simulink model "Catch_the_ball_gaming_machine"  (R2019a)
settings: Solver=VariableStepAuto  StartTime=0.0  StopTime=10.0  RelTol=1e-3
libraries: arduinolib x17
settings Model: Creator=Subhau  LastModifiedBy=Subhau

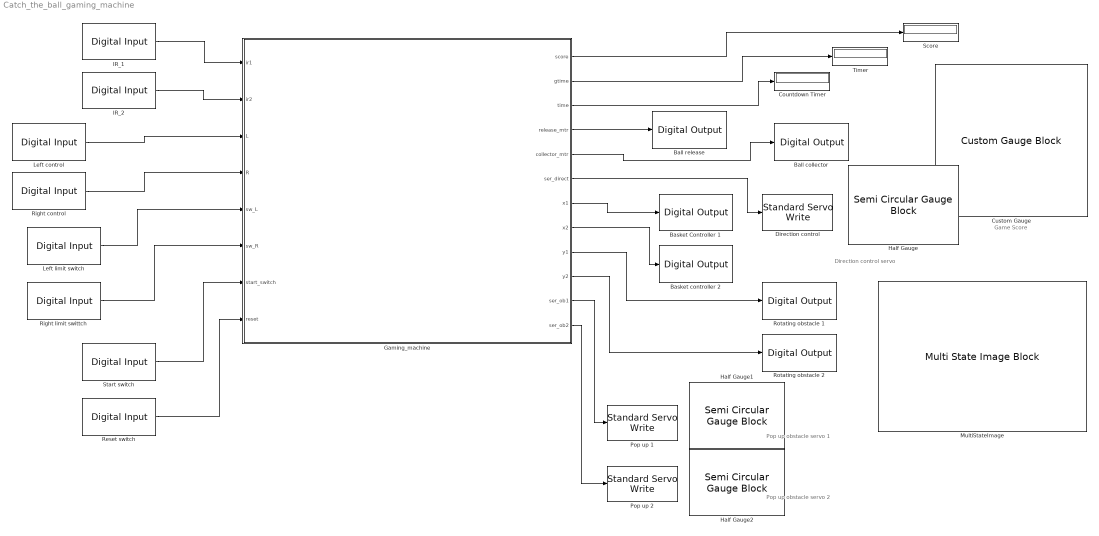
== system Catch_the_ball_gaming_machine ==
  note: Direction control servo
  note: Pop up obstacle servo 1
  note: Pop up obstacle servo 2
  note: Game Score
  Ball collector : arduinolib/Digital Output  pinNumber=20  blockPlatform=arduino
  Ball release : arduinolib/Digital Output  pinNumber=21  blockPlatform=arduino
  Basket Controller 1 : arduinolib/Digital Output  pinNumber=22  blockPlatform=arduino
  Basket controller 2 : arduinolib/Digital Output  pinNumber=23  blockPlatform=arduino
  Countdown Timer : Display
  Custom Gauge : CustomGaugeBlock  NeedleImage=data:image/svg+xml;base64,PD94bWwgdmVyc2lvbj0iMS4wIiBlbmNvZGluZz0idXRmLTgiPz4KPCEtLSBHZW5lcmF0b3I6IEFkb2JlIElsbHVzdHJhdG9yIDE5LjIuMSwgU1ZHIEV4cG9ydCBQbHVnLUluIC4gU1ZHIFZlcnNpb246IDYuMDAgQnVpbGQgMCkgIC0tPgo8c3ZnIHZlcnNpb249IjEuMSIgeG1sbnM9Imh0dHA6Ly93d3cudzMub3JnLzIwMDAvc3ZnIiB4bWxuczp4bGluaz0iaHR0cDovL3d3dy53My5vcmcvMTk5OS94bGluayIgeD0iMHB4IiB5PSIwcHgiCgkgdmlld0JveD0iMCAwIDIwMCA1MCIgc3R5bGU9ImVuYWJsZS1iYWNrZ3JvdW5kOm5ldyAw ...(+9940 chars)  NeedleXPos=0.3802298124325669  NeedleYPos=0.48117305677424654  NeedleHeight=0.11602152693163792  NeedleWidth=0.1911368983686954  NeedleInitialRotation=-59.94322499147643  BackgroundImage=data:image/svg+xml;base64,PD94bWwgdmVyc2lvbj0iMS4wIiBlbmNvZGluZz0iVVRGLTgiIHN0YW5kYWxvbmU9Im5vIj8+CjwhLS0gR2VuZXJhdG9yOiBBZG9iZSBJbGx1c3RyYXRvciAxOS4yLjEsIFNWRyBFeHBvcnQgUGx1Zy1JbiAuIFNWRyBWZXJzaW9uOiA2LjAwIEJ1aWxkIDApICAtLT4KCjxzdmcKICAgeG1sbnM6ZGM9Imh0dHA6Ly9wdXJsLm9yZy9kYy9lbGVtZW50cy8xLjEvIgogICB4bWxuczpjYz0iaHR0cDovL2NyZWF0aXZlY29tbW9ucy5vcmcvbnMjIgogICB4bWxuczpyZGY9Imh0dHA6Ly93d3cudzMub3JnLzE5OTkvMDIvMjItcmRmLXN5bnRh ...(+9660 chars)  GaugeMax=1000  GaugeArcDefined=true  GaugeArcRadius=0.1358563990074277  GaugeArcStrokeWidth=0.03972965542329953  GaugeArcRotation=240.5385250290321  GaugeArcRatio=0.8333333333333  GaugeArcTransparency=0  ValueArcColor=#1759b0  GaugeTickColor=#faf5c8  TickInterval=200  ScaleColorsJSON=[]  fixedAspectRatio=on
  Direction control : arduinolib/Standard Servo Write  pinNumber=2  ServoIndex=0  blockPlatform=ARDUINO
      settings: SourceProductName=Simulink Support Package for Arduino Hardware
  Gaming_machine : Stateflow chart  BlockKeywords=__PRM__SERIALIZED__DATA__:Stateflow Chart,Stateflow Diagram  TreatAsAtomicUnit=on
  Half Gauge : SemiCircularGaugeBlock  ScaleMax=180  TickInterval=30
  Half Gauge1 : SemiCircularGaugeBlock  ScaleMax=180  TickInterval=30
  Half Gauge2 : SemiCircularGaugeBlock  ScaleMax=180  TickInterval=30
  IR_1 : arduinolib/Digital Input  pinNumber=4  sampleTime=0.1  blockPlatform=arduino
      settings: SourceProductName=Simulink Support Package for Arduino Hardware
  IR_2 : arduinolib/Digital Input  pinNumber=5  sampleTime=0.1  blockPlatform=arduino
      settings: SourceProductName=Simulink Support Package for Arduino Hardware
  Left control : arduinolib/Digital Input  pinNumber=6  sampleTime=0.1  blockPlatform=arduino
      settings: SourceProductName=Simulink Support Package for Arduino Hardware
  Left limit switch : arduinolib/Digital Input  pinNumber=8  sampleTime=0.1  blockPlatform=arduino
      settings: SourceProductName=Simulink Support Package for Arduino Hardware
  MultiStateImage : MultiStateImageBlock
  Pop up 1 : arduinolib/Standard Servo Write  pinNumber=45  ServoIndex=1  blockPlatform=ARDUINO
      settings: SourceProductName=Simulink Support Package for Arduino Hardware
  Pop up 2 : arduinolib/Standard Servo Write  pinNumber=3  ServoIndex=2  blockPlatform=ARDUINO
      settings: SourceProductName=Simulink Support Package for Arduino Hardware
  Reset switch : arduinolib/Digital Input  pinNumber=11  sampleTime=0.1  blockPlatform=arduino
      settings: SourceProductName=Simulink Support Package for Arduino Hardware
  Right control : arduinolib/Digital Input  pinNumber=7  sampleTime=0.1  blockPlatform=arduino
      settings: SourceProductName=Simulink Support Package for Arduino Hardware
  Right limit swittch : arduinolib/Digital Input  pinNumber=9  sampleTime=0.1  blockPlatform=arduino
      settings: SourceProductName=Simulink Support Package for Arduino Hardware
  Rotating obstacle 1 : arduinolib/Digital Output  pinNumber=24  blockPlatform=arduino
  Rotating obstacle 2 : arduinolib/Digital Output  pinNumber=25  blockPlatform=arduino
  Score : Display
  Start switch : arduinolib/Digital Input  pinNumber=10  sampleTime=0.1  blockPlatform=arduino
      settings: SourceProductName=Simulink Support Package for Arduino Hardware
  Timer : Display
  wires:
  Reset switch/1 -> Gaming_machine/8(reset)
  Gaming_machine/2(gtime) -> Timer/1
  Left control/1 -> Gaming_machine/3(L)
  IR_1/1 -> Gaming_machine/1(ir1)
  Right control/1 -> Gaming_machine/4(R)
  Gaming_machine/1(score) -> Score/1
  Left limit switch/1 -> Gaming_machine/5(sw_L)
  Gaming_machine/3(time) -> Countdown Timer/1
  IR_2/1 -> Gaming_machine/2(ir2)
  Start switch/1 -> Gaming_machine/7(start_switch)
  Right limit swittch/1 -> Gaming_machine/6(sw_R)
  Gaming_machine/8(x2) -> Basket controller 2/1
  Gaming_machine/6(ser_direct) -> Direction control/1
  Gaming_machine/9(y1) -> Rotating obstacle 1/1
  Gaming_machine/4(release_mtr) -> Ball release/1
  Gaming_machine/11(ser_ob1) -> Pop up 1/1
  Gaming_machine/12(ser_ob2) -> Pop up 2/1
  Gaming_machine/7(x1) -> Basket Controller 1/1
  Gaming_machine/5(collector_mtr) -> Ball collector/1
  Gaming_machine/10(y2) -> Rotating obstacle 2/1

== stateflow chart Catch_the_ball_gaming_machine/Gaming_machine ==
  state Game_ON
    collector_mtr=1;
    release_mtr=1;
    state Game_time [parallel]
      settings: executionOrder=1
      state Time1
        gtime=gtime;
      state Time2
        gtime=gtime;
      (default) -> Game_ON.Game_time.Time1
      Game_ON.Game_time.Time2 -> Game_ON.Game_time.Time1 : [after(1,sec)&&gtime>0]{gtime = gtime - 1}
      Game_ON.Game_time.Time1 -> Game_ON.Game_time.Time2 : [after(1,sec)&&gtime>0]{gtime = gtime - 1}
    state Scoring [parallel]
      settings: executionOrder=6
      state default
        score=0;
      state dummy1
        score=score;
      state dummy2
        score=score;
      (default) -> default
      default -> dummy1
      dummy1 -> dummy2 : [ir1==1||ir2==1]{score=score+10}
      dummy2 -> dummy1 : [after(200,msec)]
    state Direction_control [parallel]
      settings: executionOrder=2
      state Servo_movement1
        ser_direct=ser_direct;
      state Servo_movement2
        ser_direct=ser_direct;
      (default) -> Servo_movement1
      Servo_movement1 -> Servo_movement1 [order 2] : [after(50,msec)&&ser_direct<170]{ser_direct = ser_direct + 1}
      Servo_movement1 -> Servo_movement2 [order 1] : [ser_direct==170]
      Servo_movement2 -> Servo_movement1 [order 2] : [ser_direct==10]
      Servo_movement2 -> Servo_movement2 [order 1] : [after(50,msec)&&ser_direct>10]{ser_direct = ser_direct - 1}
    state Obstacle_rotating [parallel]
      settings: executionOrder=5
      state Initial
        y1=0;
        y2=0;
      state State_changer
        random=randi(10);
      state State1
        y1=1;
        y2=0;
      state State2
        y1=0;
        y2=1;
      (default) -> Game_ON.Obstacle_rotating.Initial
      Game_ON.Obstacle_rotating.Initial -> State_changer
      State_changer -> State1 [order 1] : [random<=5]
      State1 -> State_changer : [after(5,sec)]
      State2 -> State_changer : [after(5,sec)]
      State_changer -> State2 [order 2] : [random>5]
    state Basket_movement [parallel]
      settings: executionOrder=3
      state Rest
        x1=0;
        x2=0;
      state Right_movement
        x1=0;
        x2=1;
      state Left_movement
        x1=1;
        x2=0;
      (default) -> Rest
      Left_movement -> Rest [order 2] : [(L==0&&R==0)||(sw_L==1&&sw_R==0)]
      Rest -> Left_movement [order 2] : [L==1&&R==0]
      Rest -> Right_movement [order 1] : [R==1&&L==0]
      Right_movement -> Rest [order 2] : [(R==0&&L==0)||(sw_R==1&&sw_L==0)]
      Left_movement -> Right_movement [order 1] : [L==0&&R==1]
      Right_movement -> Left_movement [order 1] : [L==1&&R==0]
    state Obstacle_popup [parallel]
      settings: executionOrder=4
      state Initial
        t=60;
      state Servo_movement
        state movement1
          ser_ob1=ser_ob1;
          ser_ob2=ser_ob2;
        state movement2
          ser_ob1=ser_ob1;
          ser_ob2=ser_ob2;
        (default) -> movement1
        movement1 -> movement1 [order 2] : [after(1,msec)&&ser_ob1<170&&ser_ob2<170]{ser_ob1 = ser_ob1 + 1,ser_ob2 = ser_ob2 + 1}
        movement1 -> movement2 [order 1] : [ser_ob1==170&&ser_ob2==170]
        movement2 -> movement1 [order 1] : [ser_ob1==10&&ser_ob2==10]
        movement2 -> movement2 [order 2] : [after(1,msec)&&ser_ob1>10&&ser_ob2>10]{ser_ob1 = ser_ob1 - 1,ser_ob2 = ser_ob2 - 1}
      state dummy
        t=t;
      (default) -> Game_ON.Obstacle_popup.Initial
      Game_ON.Obstacle_popup.Initial -> Servo_movement
      dummy -> Servo_movement : [after(200,msec)]
      Servo_movement -> dummy : [after(10,sec)&&t>1]{t=t-3}
  state Countdown_timer
    state Time2
      time=time;
    state Time1
      time=time;
    (default) -> Countdown_timer.Time1
    Countdown_timer.Time2 -> Countdown_timer.Time1 : [after(1,sec)&&time>0]{time = time - 1}
    Countdown_timer.Time1 -> Countdown_timer.Time2 : [after(1,sec)&&time>0]{time = time - 1}
  state Initial
    time=5;
    collector_mtr=0;
    release_mtr=0;
    ser_direct=10;
    ser_ob1=10;
    ser_ob2=10;
  (default) -> Initial
  Countdown_timer -> Game_ON : [time==0]{gtime=180}
  Initial -> Countdown_timer : [start_switch==1]
  Game_ON -> Initial : [gtime==0|| reset==1]
  data: score output; gtime output; time output; release_mtr output; collector_mtr output; ser_direct output; ir1 input; ir2 input; x1 output; x2 output; y1 output; y2 output; ser_ob1 output; ser_ob2 output; L input; R input; sw_L input; sw_R input; start_switch input; random local; t local; reset input
